simulink model "buoy_FAM_sim_v1"  (R2023b)
settings: Solver=VariableStepAuto  StartTime=0.0  StopTime=60  MaxStep=0.01  RelTol=1e-3
model workspace (MAT data in the model file):
  CD_cmmt = Simulink.Parameter
  CD_cmmt.Value = 0.5
  CD_cmmt.DataType = 'auto'
  CD_cmmt.Complexity = 'real'
  CD_cmmt.Dimensions = [1 1]
  buoy_density_cmmt = Simulink.Parameter
  buoy_density_cmmt.Value = 881
  buoy_density_cmmt.Description = 'Set to match RM3 float weight of 207.6 Mg'
  buoy_density_cmmt.DataType = 'auto'
  buoy_density_cmmt.DocUnits = 'kg/m^3'
  buoy_density_cmmt.Complexity = 'real'
  buoy_density_cmmt.Dimensions = [1 1]
  buoy_height_cmmt = Simulink.Parameter
  buoy_height_cmmt.Value = 9
  buoy_height_cmmt.Description = 'Based on Sandia RM3 model'
  buoy_height_cmmt.DataType = 'auto'
  buoy_height_cmmt.DocUnits = 'm'
  buoy_height_cmmt.Complexity = 'real'
  buoy_height_cmmt.Dimensions = [1 1]
  buoy_radius_cmmt = Simulink.Parameter
  buoy_radius_cmmt.Value = 1.8
  buoy_radius_cmmt.Description = 'Based on Sandia RM3'
  buoy_radius_cmmt.DataType = 'auto'
  buoy_radius_cmmt.DocUnits = 'm'
  buoy_radius_cmmt.Complexity = 'real'
  buoy_radius_cmmt.Dimensions = [1 1]
  fluid_density = Simulink.Parameter
  fluid_density.Value = 1025
  fluid_density.DataType = 'auto'
  fluid_density.DocUnits = 'kg/m^3'
  fluid_density.Complexity = 'real'
  fluid_density.Dimensions = [1 1]
  gravity = Simulink.Parameter
  gravity.Value = 9.81
  gravity.DataType = 'auto'
  gravity.DocUnits = 'm/s^2'
  gravity.Complexity = 'real'
  gravity.Dimensions = [1 1]
  spring_const_cmmt = Simulink.Parameter
  spring_const_cmmt.Value = 1000
  spring_const_cmmt.DataType = 'auto'
  spring_const_cmmt.DocUnits = 'N/m'
  spring_const_cmmt.Complexity = 'real'
  spring_const_cmmt.Dimensions = [1 1]
  spring_unstretched_length = Simulink.Parameter
  spring_unstretched_length.Value = -4
  spring_unstretched_length.Description = 'Value of x where spring would have 0 force. Ex. with this set to -2, there would be 0 spring force if x=-2'
  spring_unstretched_length.DataType = 'auto'
  spring_unstretched_length.DocUnits = 'm'
  spring_unstretched_length.Complexity = 'real'
  spring_unstretched_length.Dimensions = [1 1]
  wave_amplitude_cmmt = Simulink.Parameter
  wave_amplitude_cmmt.Value = 1
  wave_amplitude_cmmt.DataType = 'auto'
  wave_amplitude_cmmt.DocUnits = 'm'
  wave_amplitude_cmmt.Complexity = 'real'
  wave_amplitude_cmmt.Dimensions = [1 1]
  wave_period_cmmt = Simulink.Parameter
  wave_period_cmmt.Value = 5
  wave_period_cmmt.DataType = 'auto'
  wave_period_cmmt.DocUnits = 's'
  wave_period_cmmt.Complexity = 'real'
  wave_period_cmmt.Dimensions = [1 1]
undefined symbols (not defined in the file): buoy_density, buoy_height, buoy_radius, CD, damping, spring_const, wave_amplitude, wave_period
libraries: FAM_lab_scale x1
settings Model: Creator=Carson  LastModifiedBy=Carson

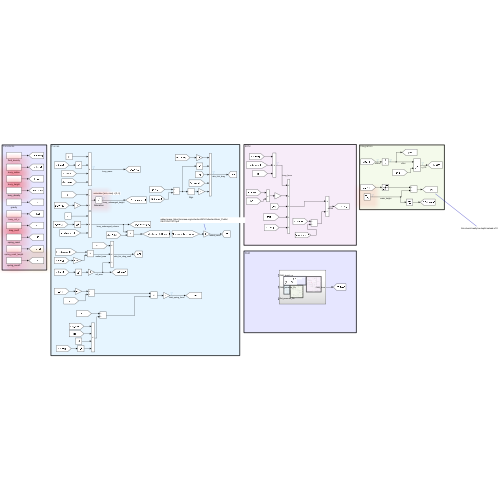
[thumbnail: Simulink's stored preview of the top-level diagram]
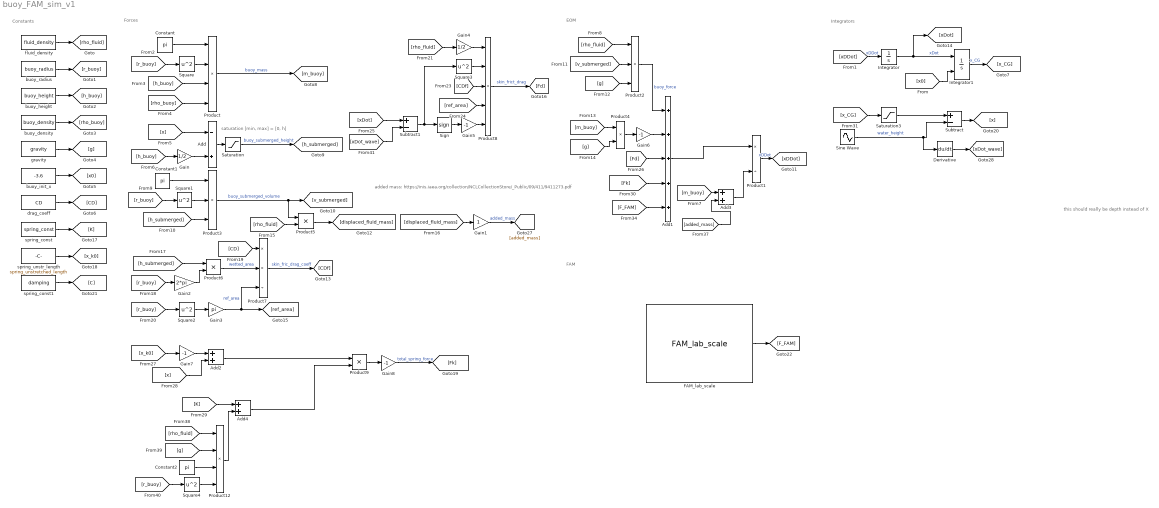
== system buoy_FAM_sim_v1 ==
  note: FAM
  note: this should really be depth instead of X
  note: EOM
  note: added mass: https://inis.iaea.org/collection/NCLCollectionStore/_Public/09/411/9411273.pdf
  note: Forces
  note: saturation [min, max] = [0, h]
  note: Integrators
  note: Constants
  Add : Sum  Inputs=-+
  Add1 : Sum  Inputs=+++++
  Add2 : Sum
  Add3 : Sum
  Add4 : Sum
  Constant : Constant  Value=pi
  Constant1 : Constant  Value=pi
  Constant2 : Constant  Value=pi
  Derivative : Derivative
  FAM_lab_scale : FAM_lab_scale/FAM_lab_scale  SystemSampleTime=-1  VariantActivationTime=update diagram  AllowFlexibleInterface=on  Latency=0  AutoFrameSizeCalculation=off
  Gain : Gain  Gain=1/2
  Gain1 : Gain
  Gain2 : Gain  Gain=2*pi
  Gain3 : Gain  Gain=pi
  Gain4 : Gain  Gain=1/2
  Gain{5..8} (4 alike) : Gain  Gain=-1
  Integrator : Integrator
  Integrator1 : Integrator  InitialConditionSource=external
  Product : Product  Inputs=****
  Product1 : Product  Inputs=*/
  Product12 : Product  Inputs=****
  Product2 : Product  Inputs=***
  Product3 : Product  Inputs=***
  Product{4..6,9} (4 alike) : Product
  Product7 : Product  Inputs=**/
  Product8 : Product  Inputs=*****
  Saturation : Saturate  UpperLimit=buoy_height  LowerLimit=0
  Saturation3 : Saturate  UpperLimit=0  LowerLimit=-100
  Sign : Signum  ZeroCross=off
  Sine Wave : Sin  Amplitude=wave_amplitude  Frequency=2*pi/wave_period  SampleTime=0
  Square{,1..4} (5 alike) : Math  Operator=square
  Subtract : Sum  Inputs=+-
  Subtract1 : Sum  Inputs=+-
  buoy_density : Constant  Value=buoy_density
  buoy_height : Constant  Value=buoy_height
  buoy_init_x : Constant  Value=-3.6
  buoy_radius : Constant  Value=buoy_radius
  drag_coeff : Constant  Value=CD
  fluid_density : Constant  Value=fluid_density
  gravity : Constant  Value=gravity
  spring_const : Constant  Value=spring_const
  spring_const1 : Constant  Value=damping
  spring_unstr_length : Constant  Value=spring_unstretched_length
  wires:
  fluid_density/1 -> [rho_fluid]
  buoy_radius/1 -> [r_buoy]
  buoy_height/1 -> [h_buoy]
  buoy_density/1 -> [rho_buoy]
  gravity/1 -> [g]
  [xDDot] -> Integrator/1  "xDDot"
  Integrator/1 -> [xDot], Integrator1/1  "xDot"
  Integrator1/1 -> [x_CG]  "x_CG"
  buoy_init_x/1 -> [x0]
  [x0] -> Integrator1/2
  Constant/1 -> Product/1
  [r_buoy] -> Square/1
  Square/1 -> Product/2
  [h_buoy] -> Product/3
  [rho_buoy] -> Product/4
  Product/1 -> [m_buoy]  "buoy_mass"
  [x] -> Add/1
  [h_buoy] -> Gain/1
  Gain/1 -> Add/2
  Saturation/1 -> [h_submerged]  "buoy_submerged_height"
  Add/1 -> Saturation/1
  Add1/1 -> Product1/1
  Product2/1 -> Add1/1  "buoy_force"
  [rho_fluid] -> Product2/1
  Square1/1 -> Product3/2
  [r_buoy] -> Square1/1
  Constant1/1 -> Product3/1
  [h_submerged] -> Product3/3
  Product3/1 -> Product5/1, [v_submerged]  "buoy_submerged_volume"
  [v_submerged] -> Product2/2
  [g] -> Product2/3
  Product4/1 -> Gain6/1
  [m_buoy] -> Product4/1
  [g] -> Product4/2
  Product1/1 -> [xDDot]  "xDDot"
  Product5/1 -> [displaced_fluid_mass]
  [rho_fluid] -> Product5/2
  [displaced_fluid_mass] -> Gain1/1
  Gain1/1 -> [added_mass]  "added_mass"
  [m_buoy] -> Add3/1
  drag_coeff/1 -> [CD]
  [h_submerged] -> Product6/1
  [r_buoy] -> Gain2/1
  Gain2/1 -> Product6/2
  Product6/1 -> Product7/2  "wetted_area"
  [CD] -> Product7/1
  [r_buoy] -> Square2/1
  Square2/1 -> Gain3/1
  Gain3/1 -> [ref_area], Product7/3  "ref_area"
  Product7/1 -> [CDf]  "skin_fric_drag_coeff"
  [rho_fluid] -> Gain4/1
  Gain4/1 -> Product8/1
  Subtract1/1 -> Square3/1, Sign/1
  Square3/1 -> Product8/2
  [CDf] -> Product8/3
  [ref_area] -> Product8/4
  Product8/1 -> [Fd]  "skin_frict_drag"
  [xDot] -> Subtract1/1
  Sign/1 -> Gain5/1
  Gain5/1 -> Product8/5
  Gain6/1 -> Add1/2
  [Fd] -> Add1/3
  spring_const/1 -> [K]
  spring_unstr_length/1 -> [x_k0]
  [x_k0] -> Gain7/1
  Gain7/1 -> Add2/1
  [x] -> Add2/2
  Add2/1 -> Product9/1
  [K] -> Add4/1
  [Fk] -> Add1/4
  Product9/1 -> Gain8/1
  Gain8/1 -> [Fk]  "total_spring_force"
  [x_CG] -> Saturation3/1
  Sine Wave/1 -> Derivative/1, Subtract/2  "water_height"
  Subtract/1 -> [x]
  spring_const1/1 -> [C]
  [F_FAM] -> Add1/5
  Saturation3/1 -> Subtract/1
  Add3/1 -> Product1/2
  [added_mass] -> Add3/2
  [rho_fluid] -> Product12/1
  Product12/1 -> Add4/2
  [g] -> Product12/2
  Constant2/1 -> Product12/3
  [r_buoy] -> Square4/1
  Square4/1 -> Product12/4
  Add4/1 -> Product9/2
  Derivative/1 -> [xDot_wave]
  [xDot_wave] -> Subtract1/2
  FAM_lab_scale/1 -> [F_FAM]
